simulink model "Lab_3_exercise1"  (R2018a)
settings: Solver=VariableStepAuto  StartTime=0.0  StopTime=8  RelTol=1e-3
values from neighbouring files (symbols this model uses):
  K = 0.5    [Lab_3_constant.m]
  T = 2    [Lab_3_constant.m]
  wn = 2    [Lab_3_constant.m]
  zeta = 3    [Lab_3_constant.m]
  zeta1 = 0.5    [Lab_3_constant.m]
  zeta2 = 0    [Lab_3_constant.m]
  zeta3 = 1    [Lab_3_constant.m]
libraries: dspsrcs4 x4, simulink x2
settings Model: Creator=WIN  LastModifiedBy=WIN

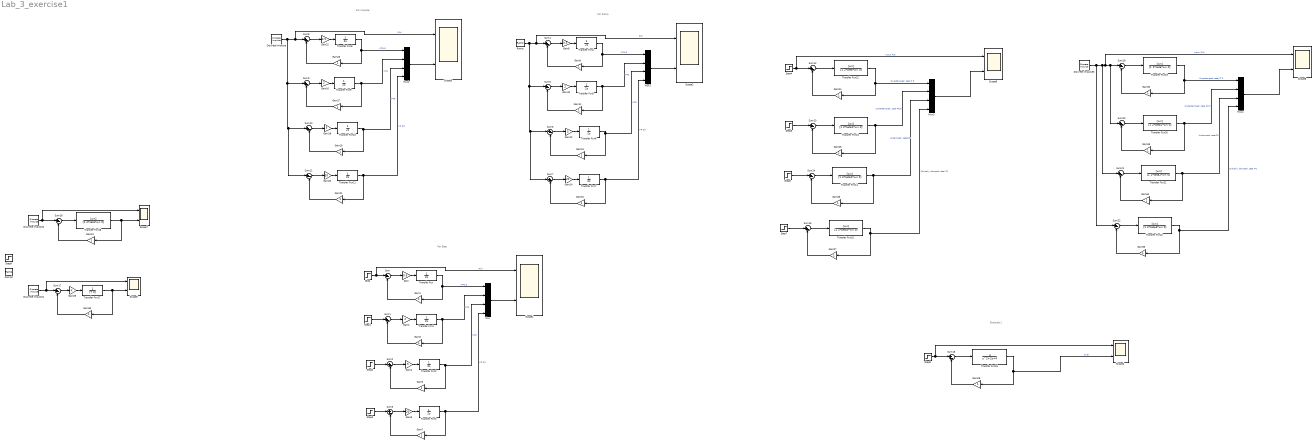
== system Lab_3_exercise1 ==
  note: Example 1
  note: For Step
  note: For Ramp
  note: For Impulse
  Discrete Impulse{,1..3} (4 alike) : dspsrcs4/Discrete  Impulse  Delay=0  SampleTime=0.1  FrameSample=1  OutputFrames=off  dataType=double  isSigned=on  wordLen=16  udDataType=sfix(16)  fracBitsMode=Best precision  numFracBits=15  OutDataTypeStr=double  LastOutDataTypeStr=double
  Gain : Gain  Gain=0.5
  Gain{1,3,5,7,9,11,13,15,17,19,21,23..28,30..35} (23 alike) : Gain
  Gain10 : Gain  Gain=2
  Gain12 : Gain  Gain=5
  Gain14 : Gain  Gain=20
  Gain16 : Gain  Gain=2
  Gain18 : Gain  Gain=5
  Gain2 : Gain  Gain=2
  Gain20 : Gain  Gain=20
  Gain22 : Gain  Gain=0.5
  Gain29 : Gain  Gain=K
  Gain4 : Gain  Gain=5
  Gain6 : Gain  Gain=20
  Gain8 : Gain  Gain=0.5
  Mux{,1..4} (5 alike) : Mux
  Ramp : simulink/Sources/Ramp  slope=1  start=0  InitialOutput=0
  Ramp2 : simulink/Sources/Ramp  slope=1  start=0  InitialOutput=0
  Scope{1..8} (8 alike) : Scope  NumInputPorts=2
  Step{,1..9} (10 alike) : Step  SampleTime=0
  Sum{,1..22} (23 alike) : Sum  Inputs=|+-
  Transfer Fcn{,1..11} (12 alike) : TransferFcn  Denominator=[2 0]
  Transfer Fcn12 : TransferFcn  Numerator=[wn]  Denominator=[1 2*zeta*wn 0]
  Transfer Fcn13 : TransferFcn  Numerator=[wn]  Denominator=[1 2*zeta1*wn 0]
  Transfer Fcn14 : TransferFcn  Numerator=[wn]  Denominator=[1 2*zeta2*wn 0]
  Transfer Fcn15 : TransferFcn  Numerator=[wn]  Denominator=[1 2*zeta3*wn 0]
  Transfer Fcn16 : TransferFcn  Numerator=[4]  Denominator=[1 2 4]
  Transfer Fcn17 : TransferFcn  Denominator=[T 0]
  Transfer Fcn18 : TransferFcn  Numerator=[wn]  Denominator=[1 2*zeta*wn 0]
  Transfer Fcn19 : TransferFcn  Numerator=[wn]  Denominator=[1 2*zeta*wn 0]
  Transfer Fcn20 : TransferFcn  Numerator=[wn]  Denominator=[1 2*zeta1*wn 0]
  Transfer Fcn21 : TransferFcn  Numerator=[wn]  Denominator=[1 2*zeta2*wn 0]
  Transfer Fcn22 : TransferFcn  Numerator=[wn]  Denominator=[1 2*zeta3*wn 0]
  wires:
  Step/1 -> Scope1/1, Sum/1  "R(s)"
  Sum/1 -> Gain/1
  Gain/1 -> Transfer Fcn/1
  Transfer Fcn/1 -> Mux/1, Gain1/1  "K=0.5"
  Gain1/1 -> Sum/2
  Gain3/1 -> Sum1/2
  Transfer Fcn1/1 -> Mux/2, Gain3/1  "K=2"
  Gain2/1 -> Transfer Fcn1/1
  Sum1/1 -> Gain2/1
  Step1/1 -> Sum1/1
  Step2/1 -> Sum2/1
  Sum2/1 -> Gain4/1
  Gain4/1 -> Transfer Fcn2/1
  Transfer Fcn2/1 -> Mux/3, Gain5/1  "K=5"
  Gain5/1 -> Sum2/2
  Gain7/1 -> Sum3/2
  Transfer Fcn3/1 -> Mux/4, Gain7/1  "K= 20"
  Gain6/1 -> Transfer Fcn3/1
  Sum3/1 -> Gain6/1
  Step3/1 -> Sum3/1
  Mux/1 -> Scope1/2
  Mux1/1 -> Scope2/2
  Sum7/1 -> Gain14/1
  Gain14/1 -> Transfer Fcn7/1
  Transfer Fcn7/1 -> Gain15/1, Mux1/4  "K= 20"
  Gain15/1 -> Sum7/2
  Gain13/1 -> Sum6/2
  Transfer Fcn6/1 -> Gain13/1, Mux1/3  "K=5"
  Gain12/1 -> Transfer Fcn6/1
  Sum6/1 -> Gain12/1
  Sum5/1 -> Gain10/1
  Gain10/1 -> Transfer Fcn5/1
  Transfer Fcn5/1 -> Gain11/1, Mux1/2  "K=2"
  Gain11/1 -> Sum5/2
  Gain9/1 -> Sum4/2
  Transfer Fcn4/1 -> Gain9/1, Mux1/1  "K=0.5"
  Gain8/1 -> Transfer Fcn4/1
  Sum4/1 -> Gain8/1
  Ramp/1 -> Sum7/1, Sum6/1, Sum5/1, Sum4/1, Scope2/1  "R(s)"
  Discrete Impulse/1 -> Scope3/1, Sum8/1, Sum9/1, Sum10/1, Sum11/1  "R(s)"
  Sum8/1 -> Gain22/1
  Gain22/1 -> Transfer Fcn8/1
  Transfer Fcn8/1 -> Mux2/1, Gain23/1  "K=0.5"
  Gain23/1 -> Sum8/2
  Gain17/1 -> Sum9/2
  Transfer Fcn9/1 -> Mux2/2, Gain17/1  "K=2"
  Gain16/1 -> Transfer Fcn9/1
  Sum9/1 -> Gain16/1
  Sum10/1 -> Gain18/1
  Gain18/1 -> Transfer Fcn10/1
  Transfer Fcn10/1 -> Mux2/3, Gain19/1  "K=5"
  Gain19/1 -> Sum10/2
  Gain21/1 -> Sum11/2
  Transfer Fcn11/1 -> Mux2/4, Gain21/1  "K= 20"
  Gain20/1 -> Transfer Fcn11/1
  Sum11/1 -> Gain20/1
  Mux2/1 -> Scope3/2
  Sum12/1 -> Transfer Fcn12/1
  Step4/1 -> Scope6/1, Sum12/1  "Input, R(s)"
  Transfer Fcn12/1 -> Mux3/1, Gain24/1  "Overdamped, zeta = 3"
  Gain24/1 -> Sum12/2
  Gain25/1 -> Sum13/2
  Transfer Fcn13/1 -> Mux3/2, Gain25/1  "Underdamped, zeta =0.5"
  Step5/1 -> Sum13/1
  Sum13/1 -> Transfer Fcn13/1
  Sum14/1 -> Transfer Fcn14/1
  Step6/1 -> Sum14/1
  Transfer Fcn14/1 -> Mux3/3, Gain26/1  "Undamped, zeta=0"
  Gain26/1 -> Sum14/2
  Gain27/1 -> Sum15/2
  Transfer Fcn15/1 -> Mux3/4, Gain27/1  "Critically damped, zeta =1"
  Step7/1 -> Sum15/1
  Sum15/1 -> Transfer Fcn15/1
  Mux3/1 -> Scope6/2
  Gain28/1 -> Sum16/2
  Transfer Fcn16/1 -> Scope4/2, Gain28/1  "Over"
  Step8/1 -> Sum16/1, Scope4/1
  Sum16/1 -> Transfer Fcn16/1
  Gain30/1 -> Sum17/2
  Transfer Fcn17/1 -> Gain30/1, Scope5/2
  Gain29/1 -> Transfer Fcn17/1
  Sum17/1 -> Gain29/1
  Discrete Impulse1/1 -> Sum17/1, Scope5/1
  Gain31/1 -> Sum18/2
  Transfer Fcn18/1 -> Gain31/1, Scope7/2
  Discrete Impulse2/1 -> Sum18/1, Scope7/1
  Sum18/1 -> Transfer Fcn18/1
  Mux4/1 -> Scope8/2
  Sum22/1 -> Transfer Fcn22/1
  Transfer Fcn22/1 -> Gain35/1, Mux4/4  "Critically damped, zeta =1"
  Gain35/1 -> Sum22/2
  Gain34/1 -> Sum21/2
  Transfer Fcn21/1 -> Gain34/1, Mux4/3  "Undamped, zeta=0"
  Sum21/1 -> Transfer Fcn21/1
  Sum20/1 -> Transfer Fcn20/1
  Transfer Fcn20/1 -> Gain33/1, Mux4/2  "Underdamped, zeta =0.5"
  Gain33/1 -> Sum20/2
  Gain32/1 -> Sum19/2
  Transfer Fcn19/1 -> Gain32/1, Mux4/1  "Overdamped, zeta = 3"
  Discrete Impulse3/1 -> Sum22/1, Sum21/1, Sum20/1, Sum19/1, Scope8/1  "Input, R(s)"
  Sum19/1 -> Transfer Fcn19/1
